simulink model "vehicle_dynamics_turning"  (R2020a)
settings: Solver=VariableStepAuto  StartTime=0.0  StopTime=10  FixedStep=0.001  RelTol=1e-5
values from neighbouring files (symbols this model uses):
  Caf = 1290    [aa_main_code.m]    (also in aa_main_code_optimization.m)
  Car = 3000    [aa_main_code.m]    (also in aa_main_code_optimization.m)
  CG_a = (mass_x_dis/mass_CG) - L104    [aa_main_code.m]    (also in aa_main_code_optimization.m)
  CG_b = L101 - CG_a    [aa_main_code.m]    (also in aa_main_code_optimization.m)
  Cmzf = 30    [aa_main_code.m]    (also in aa_main_code_optimization.m)
  Cmzr = 20    [aa_main_code.m]    (also in aa_main_code_optimization.m)
  enablePlotting = false    [aa_main_code.m]    (also in aa_main_code_optimization.m)
  Jz = 2380    [aa_main_code.m]    (also in aa_main_code_optimization.m)
  mass = (4*passenger_mass)+cargo_mass+info_mass+sunroof_mass+unsprung_mass+total_gearbox_mass+total_differential_mass+axle_mass+body_mass+frame_rail_mass+battery_mass+total_motorinverter_mass    (= 1622.8836992)    [aa_main_code.m]    (also in aa_main_code_optimization.m = (4*passenger_mass)+cargo_mass+info_mass+sunroof_mass+unsprun)
  maxYawRate = 20    [aa_main_code.m]    (also in aa_main_code_optimization.m)
  steerAngle = 6    [aa_main_code.m]    (also in aa_main_code_optimization.m = 10)
  steeringScenario = 1    [aa_main_code.m]    (also in aa_main_code_optimization.m)
  V = V-0.5    (= 30)    [aa_main_code.m]    (also in aa_main_code_optimization.m = 39)
libraries: aerolibconvert2 x2, simulink x2, simulink_extras x2, vehdynlibviscommon x1
settings Model: Creator=SVIRK  LastModifiedBy=atefe
settings DebuggingCC: AlgebraicLoopMsg=none

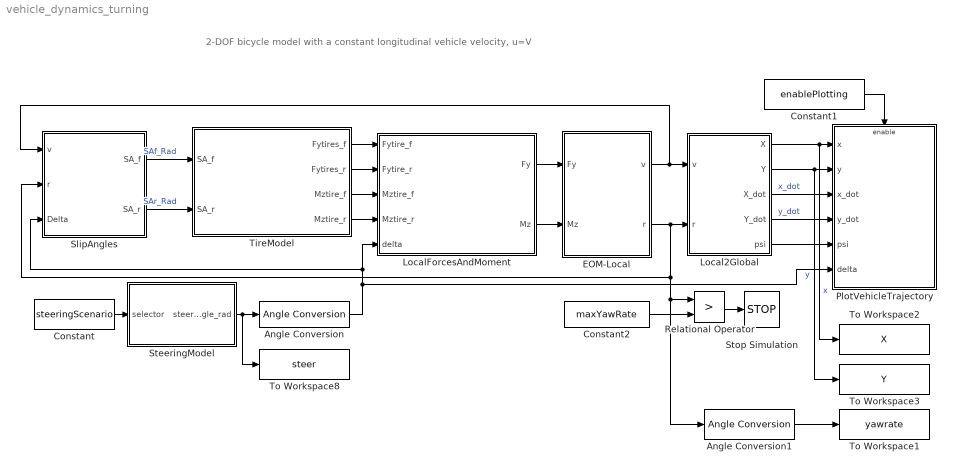
== system vehicle_dynamics_turning ==
  note: 2-DOF bicycle model with a constant longitudinal vehicle velocity, u=V
  Angle Conversion : aerolibconvert2/Angle Conversion  IU=deg  OU=rad
  Angle Conversion1 : aerolibconvert2/Angle Conversion  IU=rad  OU=deg
  Constant : Constant  Value=steeringScenario
  Constant1 : Constant  Value=enablePlotting
  Constant2 : Constant  Value=maxYawRate
  EOM-Local : Subsystem
  Local2Global : Subsystem
  LocalForcesAndMoment : Subsystem
  PlotVehicleTrajectory : Subsystem
  Relational Operator : RelationalOperator  Operator=>  OutDataTypeStr=boolean  RndMeth=Simplest
  SlipAngles : Subsystem
  SteeringModel : Subsystem
  Stop Simulation : Stop
  TireModel : Subsystem
  To Workspace1 : ToWorkspace  VariableName=yawrate  SaveFormat=Timeseries  SampleTime=-1
  To Workspace2 : ToWorkspace  VariableName=X  SaveFormat=Timeseries  SampleTime=-1
  To Workspace3 : ToWorkspace  VariableName=Y  SaveFormat=Timeseries  SampleTime=-1
  To Workspace8 : ToWorkspace  VariableName=steer  SaveFormat=Timeseries  SampleTime=-1
  wires:
  Angle Conversion/1 -> PlotVehicleTrajectory/6(delta), SlipAngles/3(Delta), LocalForcesAndMoment/5(delta)
  SlipAngles/1(SA_f) -> TireModel/1(SA_f)  "SAf_Rad"
  SlipAngles/2(SA_r) -> TireModel/2(SA_r)  "SAr_Rad"
  TireModel/1(Fytires_f) -> LocalForcesAndMoment/1(Fytire_f)
  TireModel/2(Fytires_r) -> LocalForcesAndMoment/2(Fytire_r)
  TireModel/3(Mztire_f) -> LocalForcesAndMoment/3(Mztire_f)
  TireModel/4(Mztire_r) -> LocalForcesAndMoment/4(Mztire_r)
  LocalForcesAndMoment/1(Fy) -> EOM-Local/1(Fy)
  LocalForcesAndMoment/2(Mz) -> EOM-Local/2(Mz)
  Local2Global/1(X) -> PlotVehicleTrajectory/1(x), To Workspace2/1  "x"
  Local2Global/2(Y) -> PlotVehicleTrajectory/2(y), To Workspace3/1  "y"
  Local2Global/3(X_dot) -> PlotVehicleTrajectory/3(x_dot)  "x_dot"
  Local2Global/4(Y_dot) -> PlotVehicleTrajectory/4(y_dot)  "y_dot"
  SteeringModel/1(steerAngle_rad) -> To Workspace8/1, Angle Conversion/1
  Constant/1 -> SteeringModel/1(selector)
  Local2Global/5(psi) -> PlotVehicleTrajectory/5(psi)
  Constant1/1 -> PlotVehicleTrajectory/Enable
  Constant2/1 -> Relational Operator/2
  Relational Operator/1 -> Stop Simulation/1
  Angle Conversion1/1 -> To Workspace1/1
  EOM-Local/1(v) -> Local2Global/1(v), SlipAngles/1(v)
  EOM-Local/2(r) -> Local2Global/2(r), Relational Operator/1, Angle Conversion1/1, SlipAngles/2(r)

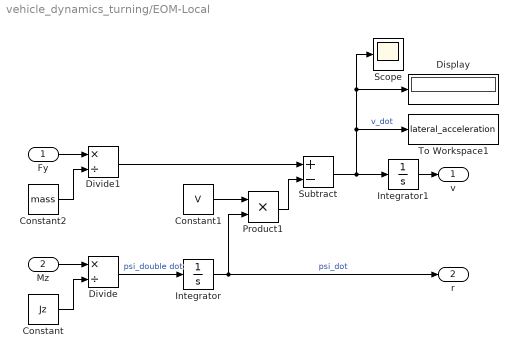
== system vehicle_dynamics_turning/EOM-Local ==
  Fy : Inport
  Mz : Inport  Port=2
  Constant : Constant  Value=Jz
  Constant1 : Constant  Value=V
  Constant2 : Constant  Value=mass
  Display : Display
  Divide : Product  Inputs=*/
  Divide1 : Product  Inputs=*/
  Integrator : Integrator
  Integrator1 : Integrator
  Product1 : Product
  Scope : Scope
  Subtract : Sum  Inputs=+-
  To Workspace1 : ToWorkspace  VariableName=lateral_acceleration  SaveFormat=Timeseries  SampleTime=-1
  v : Outport
  r : Outport  Port=2
  wires:
  Fy/1 -> Divide1/1
  Mz/1 -> Divide/1
  Integrator/1 -> Product1/2, r/1  "psi_dot"
  Constant/1 -> Divide/2
  Divide/1 -> Integrator/1  "psi_double dot"
  Divide1/1 -> Subtract/1
  Product1/1 -> Subtract/2
  Integrator1/1 -> v/1
  Subtract/1 -> Integrator1/1, Display/1, Scope/1, To Workspace1/1  "v_dot"
  Constant1/1 -> Product1/1
  Constant2/1 -> Divide1/2

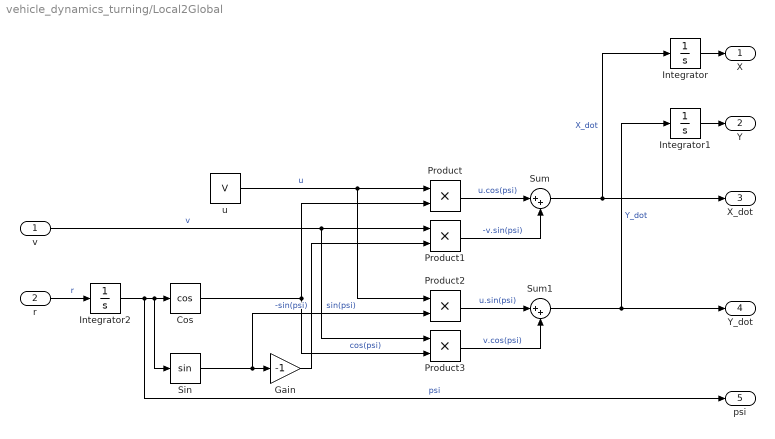
== system vehicle_dynamics_turning/Local2Global ==
  v : Inport
  r : Inport  Port=2
  Cos : Trigonometry  Operator=cos
  Gain : Gain  Gain=-1
  Integrator : Integrator
  Integrator1 : Integrator
  Integrator2 : Integrator
  Product{,1..3} (4 alike) : Product
  Sin : Trigonometry
  Sum : Sum  Inputs=|++
  Sum1 : Sum  Inputs=|++
  u : Constant  Value=V
  X : Outport
  Y : Outport  Port=2
  X_dot : Outport  Port=3
  Y_dot : Outport  Port=4
  psi : Outport  Port=5
  wires:
  Integrator1/1 -> Y/1
  Integrator/1 -> X/1
  Integrator2/1 -> Cos/1, Sin/1, psi/1  "psi"
  Sum/1 -> Integrator/1, X_dot/1  "X_dot"
  u/1 -> Product/1, Product2/1  "u"
  Cos/1 -> Product3/2, Product/2  "cos(psi)"
  Sin/1 -> Product2/2, Gain/1  "sin(psi)"
  Gain/1 -> Product1/2  "-sin(psi)"
  v/1 -> Product1/1, Product3/1  "v"
  Product/1 -> Sum/1  "u.cos(psi)"
  Product1/1 -> Sum/2  "-v.sin(psi)"
  Product2/1 -> Sum1/1  "u.sin(psi)"
  Product3/1 -> Sum1/2  "v.cos(psi)"
  Sum1/1 -> Integrator1/1, Y_dot/1  "Y_dot"
  r/1 -> Integrator2/1  "r"

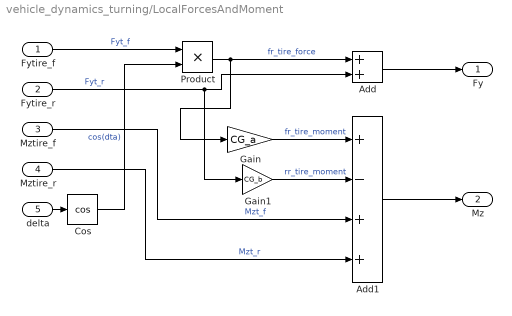
== system vehicle_dynamics_turning/LocalForcesAndMoment ==
  Fytire_f : Inport
  Fytire_r : Inport  Port=2
  Mztire_f : Inport  Port=3
  Mztire_r : Inport  Port=4
  delta : Inport  Port=5
  Add : Sum
  Add1 : Sum  Inputs=+-++
  Cos : Trigonometry  Operator=cos
  Gain : Gain  Gain=CG_a
  Gain1 : Gain  Gain=CG_b
  Product : Product
  Fy : Outport
  Mz : Outport  Port=2
  wires:
  Fytire_r/1 -> Gain1/1, Add/2  "Fyt_r"
  Fytire_f/1 -> Product/1  "Fyt_f"
  Mztire_r/1 -> Add1/4  "Mzt_r"
  delta/1 -> Cos/1
  Mztire_f/1 -> Add1/3  "Mzt_f"
  Cos/1 -> Product/2  "cos(dta)"
  Product/1 -> Gain/1, Add/1  "fr_tire_force"
  Gain/1 -> Add1/1  "fr_tire_moment"
  Gain1/1 -> Add1/2  "rr_tire_moment"
  Add/1 -> Fy/1
  Add1/1 -> Mz/1

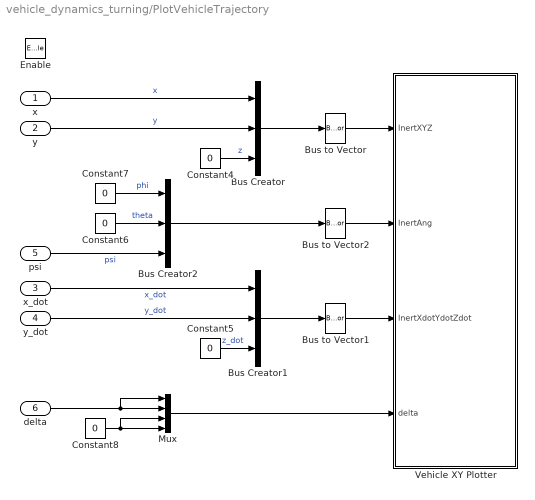
== system vehicle_dynamics_turning/PlotVehicleTrajectory ==
  x : Inport
  y : Inport  Port=2
  x_dot : Inport  Port=3
  y_dot : Inport  Port=4
  psi : Inport  Port=5
  delta : Inport  Port=6
  Enable : EnablePort
  Bus Creator : BusCreator  Inputs=3
  Bus Creator1 : BusCreator  Inputs=3
  Bus Creator2 : BusCreator  Inputs=3
  Bus to Vector : BusToVector
  Bus to Vector1 : BusToVector
  Bus to Vector2 : BusToVector
  Constant{4..8} (5 alike) : Constant  Value=0
  Mux : Mux
  Vehicle XY Plotter : Subsystem  mask(Vehicle XY Plotter){a=CG_a, b=CG_b, w=1.5, figBorder=5, bufferSize=1024, extRef=off, pltDT=.1}
      mask prompts: a "Distance to front axle from CG, a [m]:"; b "Distance to rear axle from CG, b [m]:"; w "Track width, w [m]:"; figBorder "Distance to figure borders, figBorder [m]:"; bufferSize "Path buffer sampe size, bufferSize []:"; extRef "Plot path reference, extRef"; pltDT "Plot update rate, pltDT [s]:"
      mask help:
      | This block will display a MATLAB figure which indicates the vehicle path, current position and heading velocity.
      | An optional path reference is also provided.
      mask init:
      | if autoblkschecksimstopped(gcb)
      |     PortName = 'RefXYZ';
      |     InportOption  = {'built-in/Ground', [PortName, ' Ground'];...
      |         'built-in/Inport',PortName };
      |     if ~strcmp(get_param(gcb,'extRef'),'on')
      |         NewBlkHdl = autoblksreplaceblock(gcb, InportOption, 1);
      |         set_param(NewBlkHdl, 'ShowName', 'off');
      |     else
      |         autoblksreplaceblock(gcb, InportOption, 2);
      |     end
      | end
      mask TypeOptions a: Vehicle XY Plotter/a
      mask TypeOptions b: Vehicle XY Plotter/b
      mask TypeOptions w: Vehicle XY Plotter/w
      mask TypeOptions figBorder: Vehicle XY Plotter/figBorder
      mask TypeOptions bufferSize: Vehicle XY Plotter/bufferSize
  wires:
  Bus Creator1/1 -> Bus to Vector1/1
  Constant7/1 -> Bus Creator2/1  "phi"
  Constant6/1 -> Bus Creator2/2  "theta"
  Constant4/1 -> Bus Creator/3  "z"
  Constant5/1 -> Bus Creator1/3  "z_dot"
  Bus Creator2/1 -> Bus to Vector2/1
  Bus to Vector2/1 -> Vehicle XY Plotter/2(InertAng)
  y_dot/1 -> Bus Creator1/2  "y_dot"
  Bus Creator/1 -> Bus to Vector/1
  Bus to Vector1/1 -> Vehicle XY Plotter/3(InertXdotYdotZdot)
  Bus to Vector/1 -> Vehicle XY Plotter/1(InertXYZ)
  y/1 -> Bus Creator/2  "y"
  x/1 -> Bus Creator/1  "x"
  x_dot/1 -> Bus Creator1/1  "x_dot"
  Mux/1 -> Vehicle XY Plotter/4(delta)
  Constant8/1 -> Mux/3, Mux/4
  delta/1 -> Mux/1, Mux/2
  psi/1 -> Bus Creator2/3  "psi"

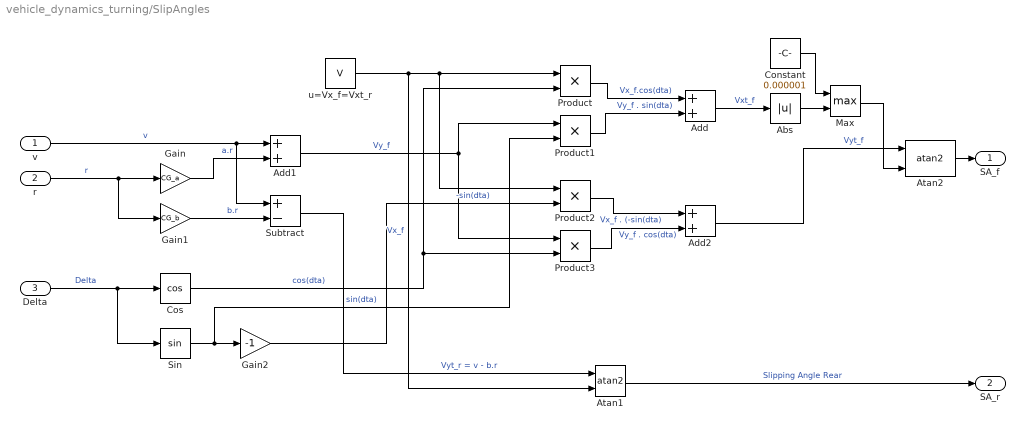
== system vehicle_dynamics_turning/SlipAngles ==
  v : Inport
  r : Inport  Port=2
  Delta : Inport  Port=3
  Abs : Abs
  Add : Sum
  Add1 : Sum
  Add2 : Sum
  Atan1 : Trigonometry  Operator=atan2
  Atan2 : Trigonometry  Operator=atan2
  Constant : Constant  Value=0.000001
  Cos : Trigonometry  Operator=cos
  Gain : Gain  Gain=CG_a
  Gain1 : Gain  Gain=CG_b
  Gain2 : Gain  Gain=-1
  Max : MinMax  Function=max  Inputs=2
  Product{,1..3} (4 alike) : Product
  Sin : Trigonometry
  Subtract : Sum  Inputs=+-
  u=Vx_f=Vxt_r : Constant  Value=V
  SA_f : Outport
  SA_r : Outport  Port=2
  wires:
  v/1 -> Add1/1, Subtract/1  "v"
  r/1 -> Gain1/1, Gain/1  "r"
  Delta/1 -> Sin/1, Cos/1  "Delta"
  Atan2/1 -> SA_f/1
  Gain/1 -> Add1/2  "a.r"
  Add1/1 -> Product1/1, Product3/1  "Vy_f"
  Sin/1 -> Product1/2, Gain2/1  "sin(dta)"
  Gain2/1 -> Product2/2  "-sin(dta)"
  Cos/1 -> Product3/2, Product/2  "cos(dta)"
  u=Vx_f=Vxt_r/1 -> Atan1/2, Product/1, Product2/1  "Vx_f"
  Product/1 -> Add/1  "Vx_f.cos(dta)"
  Product1/1 -> Add/2  "Vy_f . sin(dta)"
  Product2/1 -> Add2/1  "Vx_f . (-sin(dta)"
  Product3/1 -> Add2/2  "Vy_f . cos(dta)"
  Gain1/1 -> Subtract/2  "b.r"
  Subtract/1 -> Atan1/1  "Vyt_r = v - b.r"
  Atan1/1 -> SA_r/1  "Slipping Angle Rear"
  Add2/1 -> Atan2/1  "Vyt_f"
  Add/1 -> Abs/1  "Vxt_f"
  Abs/1 -> Max/2
  Constant/1 -> Max/1
  Max/1 -> Atan2/2

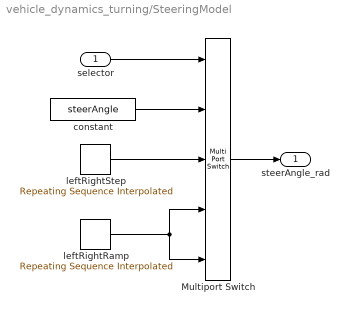
== system vehicle_dynamics_turning/SteeringModel ==
  selector : Inport
  Multiport Switch : MultiPortSwitch  DataPortForDefault=Additional data port  DiagnosticForDefault=Warning
  constant : Constant  Value=steerAngle
  leftRightRamp : simulink/Sources/Repeating Sequence Interpolated  OutValues=[0 steerAngle -steerAngle 0 0].'  TimeValues=[0 0.5 1.5 2 100].'  LookUpMeth=Interpolation-Use End Values  tsamp=0.01  OutMin=[]  OutMax=[]  OutDataTypeStr=double  OutputDataTypeScalingMode=double  OutDataType=fixdt(0,8)  OutScaling=2^-10
  leftRightStep : simulink/Sources/Repeating Sequence Interpolated  OutValues=[steerAngle steerAngle -steerAngle -steerAngle -1 -1].'  TimeValues=[0 1 1+1e-10 2 2+1e-10 100].'  LookUpMeth=Interpolation-Use End Values  tsamp=0.01  OutMin=[]  OutMax=[]  OutDataTypeStr=double  OutputDataTypeScalingMode=double  OutDataType=fixdt(0,8)  OutScaling=2^-10
  steerAngle_rad : Outport
  wires:
  leftRightRamp/1 -> Multiport Switch/5, Multiport Switch/4
  leftRightStep/1 -> Multiport Switch/3
  constant/1 -> Multiport Switch/2
  Multiport Switch/1 -> steerAngle_rad/1
  selector/1 -> Multiport Switch/1

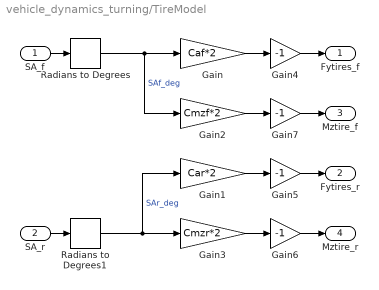
== system vehicle_dynamics_turning/TireModel ==
  SA_f : Inport
  SA_r : Inport  Port=2
  Gain : Gain  Gain=Caf*2
  Gain1 : Gain  Gain=Car*2
  Gain2 : Gain  Gain=Cmzf*2
  Gain3 : Gain  Gain=Cmzr*2
  Gain{4..7} (4 alike) : Gain  Gain=-1
  Radians to Degrees : simulink_extras/Transformations/Radians to Degrees
  Radians to Degrees1 : simulink_extras/Transformations/Radians to Degrees
  Fytires_f : Outport
  Fytires_r : Outport  Port=2
  Mztire_f : Outport  Port=3
  Mztire_r : Outport  Port=4
  wires:
  Radians to Degrees/1 -> Gain2/1, Gain/1  "SAf_deg"
  Radians to Degrees1/1 -> Gain1/1, Gain3/1  "SAr_deg"
  SA_f/1 -> Radians to Degrees/1
  SA_r/1 -> Radians to Degrees1/1
  Gain/1 -> Gain4/1
  Gain4/1 -> Fytires_f/1
  Gain1/1 -> Gain5/1
  Gain5/1 -> Fytires_r/1
  Gain3/1 -> Gain6/1
  Gain2/1 -> Gain7/1
  Gain6/1 -> Mztire_r/1
  Gain7/1 -> Mztire_f/1

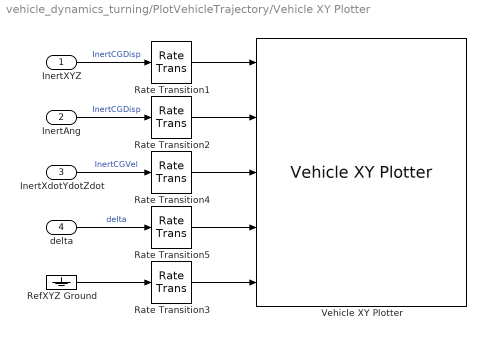
== system vehicle_dynamics_turning/PlotVehicleTrajectory/Vehicle XY Plotter ==
  InertXYZ : Inport
  InertAng : Inport  Port=2
  InertXdotYdotZdot : Inport  Port=3
  delta : Inport  Port=4
  Rate Transition{1..5} (5 alike) : RateTransition  Deterministic=off  OutPortSampleTime=pltDT
  RefXYZ Ground : Ground
  Vehicle XY Plotter : vehdynlibviscommon/Vehicle XY Plotter  bufferSize=bufferSize  w=w  a=a  b=b  figBorder=figBorder
      settings: SourceProductBaseCode=VE
  wires:
  InertAng/1 -> Rate Transition2/1  "InertCGDisp"
  InertXdotYdotZdot/1 -> Rate Transition4/1  "InertCGVel"
  InertXYZ/1 -> Rate Transition1/1  "InertCGDisp"
  delta/1 -> Rate Transition5/1  "delta"
  Rate Transition3/1 -> Vehicle XY Plotter/5
  Rate Transition1/1 -> Vehicle XY Plotter/1
  Rate Transition2/1 -> Vehicle XY Plotter/2
  Rate Transition4/1 -> Vehicle XY Plotter/3
  Rate Transition5/1 -> Vehicle XY Plotter/4
  RefXYZ Ground/1 -> Rate Transition3/1
